simulink model "Robotica"  (R2016b)
settings: Solver=ode45  StartTime=0.0  StopTime=10.0  RelTol=1e-3  EnableMultiTasking=on
libraries: vrlib x1
settings Model: Creator=David  LastModifiedBy=Didi
settings DataIOCC: LimitDataPoints=on  SaveFormat=Array
settings OptimizationCC: LifeSpan=inf
settings DebuggingCC: SFUnexpectedBacktrackingDiag=warning  SFNoUnconditionalDefaultTransitionDiag=warning  SFExecutionAtInitializationDiag=none
settings HardwareCC: ProdBitPerPointer=32  ProdBitPerSizeT=32  ProdBitPerPtrDiffT=32  ProdLargestAtomicFloat=None  ProdIntDivRoundTo=Undefined  ProdEndianess=Unspecified  ProdWordSize=32  ProdHWDeviceType=32-bit Generic
settings ModelReferenceCC: PropagateSignalLabelsOutOfModel=off
settings GRTTargetCC: TargetLangStandard=C89/C90 (ANSI)  GeneratePreprocessorConditionals=Disable all
settings ConfigComp: CovMetricSettings=dw  CovHtmlReporting=on  CovSaveCumulativeToWorkspaceVar=on  CovSaveSingleToWorkspaceVar=on  CovExternalEMLEnable=off

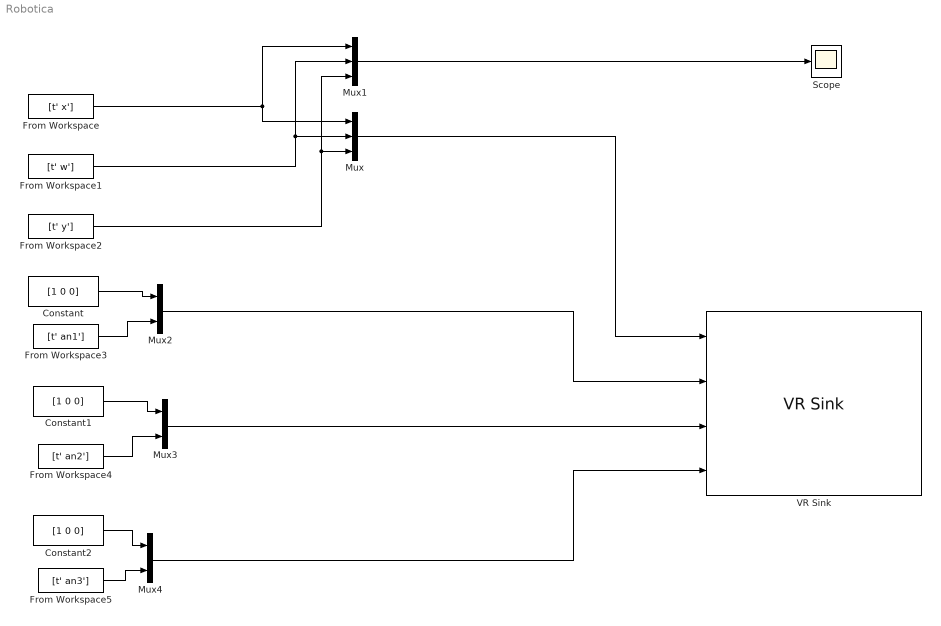
== system Robotica ==
  Constant : Constant  Value=[1 0 0]
  Constant1 : Constant  Value=[1 0 0]
  Constant2 : Constant  Value=[1 0 0]
  From Workspace : FromWorkspace  VariableName=[t' x']  SampleTime=0
  From Workspace1 : FromWorkspace  VariableName=[t' w']  SampleTime=0
  From Workspace2 : FromWorkspace  VariableName=[t' y']  SampleTime=0
  From Workspace3 : FromWorkspace  VariableName=[t' an1']  SampleTime=0
  From Workspace4 : FromWorkspace  VariableName=[t' an2']  SampleTime=0
  From Workspace5 : FromWorkspace  VariableName=[t' an3']  SampleTime=0
  Mux : Mux  Inputs=3
  Mux1 : Mux  Inputs=3
  Mux2 : Mux  Inputs=2
  Mux3 : Mux  Inputs=2
  Mux4 : Mux  Inputs=2
  Scope : Scope
  VR Sink : vrlib/VR Sink  InstantiateOnLoad=on  SampleTime=0.01  ViewEnable=on  RemoteChange=off  RemoteView=off  FieldsWritten=base.translation.3.1.1.double#rueda1.rotation.4.1.1.double#rueda2.rotation.4.1.1.double#rueda3.rotation.4.1.1.double  WorldFileName=Omnidir.WRL  AutoView=off  VideoDimensions=[]  AllowVariableSize=off
  wires:
  From Workspace/1 -> Mux1/1, Mux/1
  From Workspace1/1 -> Mux1/2, Mux/2
  From Workspace2/1 -> Mux1/3, Mux/3
  Mux1/1 -> Scope/1
  Constant/1 -> Mux2/1
  From Workspace3/1 -> Mux2/2
  Constant1/1 -> Mux3/1
  From Workspace4/1 -> Mux3/2
  Constant2/1 -> Mux4/1
  From Workspace5/1 -> Mux4/2
  Mux2/1 -> VR Sink/2
  Mux3/1 -> VR Sink/3
  Mux4/1 -> VR Sink/4
  Mux/1 -> VR Sink/1
